simulink model "HybridEVModel"  (R2024b)
settings: Solver=ode45  StartTime=0.0  StopTime=421200  RelTol=1e-3
settings Model: Creator=zs  LastModifiedBy=zs
settings DataIOCC: SaveState=on

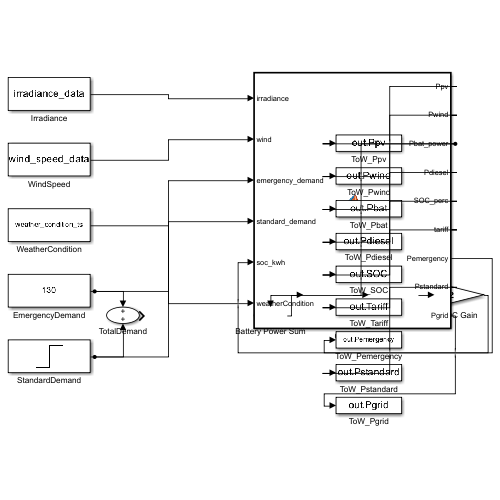
[thumbnail: Simulink's stored preview of the top-level diagram]
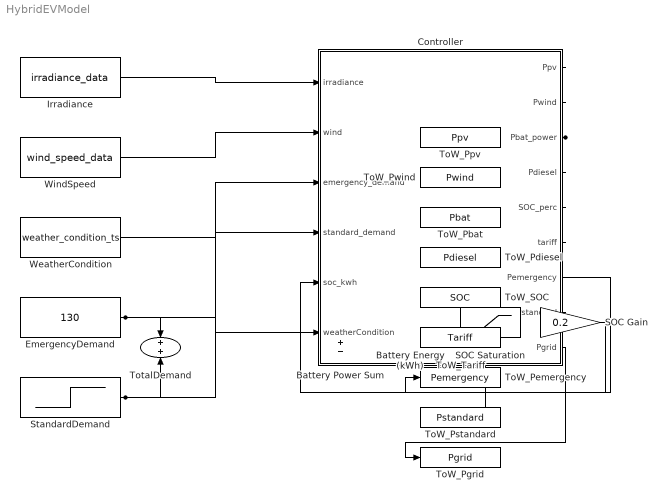
== system HybridEVModel ==
  Battery Energy (kWh) : Integrator  InitialCondition=250
  Battery Power Sum : Sum  Inputs=+-
  Controller : MATLAB Function  TreatAsAtomicUnit=on
  EmergencyDemand : Constant  Value=130
  Irradiance : FromWorkspace  VariableName=irradiance_data
  SOC Gain : Gain  Gain=0.2
  SOC Saturation : Saturate  UpperLimit=500  LowerLimit=0
  StandardDemand : Step  Time=28800  Before=1170  After=1170  SampleTime=0
  ToW_Pbat : ToWorkspace  VariableName=Pbat  SaveFormat=Timeseries  SampleTime=-1
  ToW_Pdiesel : ToWorkspace  VariableName=Pdiesel  SaveFormat=Timeseries  SampleTime=-1
  ToW_Pemergency : ToWorkspace  VariableName=Pemergency  SaveFormat=Timeseries  SampleTime=-1
  ToW_Pgrid : ToWorkspace  VariableName=Pgrid  SaveFormat=Timeseries  SampleTime=-1
  ToW_Ppv : ToWorkspace  VariableName=Ppv  SaveFormat=Timeseries  SampleTime=-1
  ToW_Pstandard : ToWorkspace  VariableName=Pstandard  SaveFormat=Timeseries  SampleTime=-1
  ToW_Pwind : ToWorkspace  VariableName=Pwind  SaveFormat=Timeseries  SampleTime=-1
  ToW_SOC : ToWorkspace  VariableName=SOC  SaveFormat=Timeseries  SampleTime=-1
  ToW_Tariff : ToWorkspace  VariableName=Tariff  SaveFormat=Timeseries  SampleTime=-1
  TotalDemand : Sum
  WeatherCondition : FromWorkspace  VariableName=weather_condition_ts
  WindSpeed : FromWorkspace  VariableName=wind_speed_data
  wires:
  Irradiance/1 -> Controller/1(irradiance)
  WindSpeed/1 -> Controller/2(wind)
  WeatherCondition/1 -> Controller/6(weatherCondition)
  EmergencyDemand/1 -> TotalDemand/1, Controller/3(emergency_demand)
  StandardDemand/1 -> TotalDemand/2, Controller/4(standard_demand)
  Controller/1(Ppv) -> ToW_Ppv/1
  Controller/2(Pwind) -> ToW_Pwind/1
  Controller/3(Pbat_power) -> ToW_Pbat/1, Battery Power Sum/1
  Controller/4(Pdiesel) -> ToW_Pdiesel/1
  Controller/5(SOC_perc) -> ToW_SOC/1
  Controller/6(tariff) -> ToW_Tariff/1
  Controller/7(Pemergency) -> ToW_Pemergency/1
  Controller/8(Pstandard) -> ToW_Pstandard/1
  Controller/9(Pgrid) -> ToW_Pgrid/1
  Battery Power Sum/1 -> Battery Energy (kWh)/1
  Battery Energy (kWh)/1 -> SOC Saturation/1
  SOC Saturation/1 -> SOC Gain/1
  SOC Gain/1 -> Controller/5(soc_kwh)

== matlab function HybridEVModel/Controller ==
  data: irradiance input; Ppv output; wind input; emergency_demand input; standard_demand input; soc_kwh input; weatherCondition input; Pwind output; Pbat_power output; Pdiesel output; SOC_perc output; tariff output; Pemergency output; Pstandard output; Pgrid output
function [Ppv, Pwind, Pbat_power, Pdiesel, SOC_perc, tariff, Pemergency, Pstandard, Pgrid] = fcn(irradiance, wind, emergency_demand, standard_demand, soc_kwh, weatherCondition)
Ppv = 0; Pwind = 0; Pbat_power = 0; Pdiesel = 0;
Pemergency = 0; Pstandard = 0; Pgrid = 0;
tariff = 0.30;
SOC_perc = 50;

panel_area = 300; solar_eff = 0.18;
rotor_diameter = 50; rho = 1.225; cp = 0.4;
rotor_area = pi * (rotor_diameter/2)^2;

if weatherCondition == 0
    solar_eff = solar_eff * 0.7;
    cp = cp * 0.8;
elseif weatherCondition == 2
    solar_eff = solar_eff * 1.2;
    cp = cp * 1.1;
end

Ppv = irradiance * panel_area * solar_eff / 1000;
Pwind = 0.5 * rho * rotor_area * (wind^3) * cp / 1000;
P_total = Ppv + Pwind;

battery_capacity = 500;
charge_eff = 0.95;
discharge_eff = 0.95;
diesel_min_soc = 0.2;

if P_total >= emergency_demand
    Pemergency = emergency_demand;
    excess = (P_total - emergency_demand) * charge_eff;
    soc_kwh = min(battery_capacity, soc_kwh + excess);
else
    Pemergency = P_total;
    remaining_emergency = emergency_demand - P_total;
    
    if soc_kwh >= remaining_emergency / discharge_eff
        Pemergency = Pemergency + remaining_emergency;
        soc_kwh = soc_kwh - (remaining_emergency / discharge_eff);
    else
        available_from_battery = soc_kwh * discharge_eff;
        Pemergency = Pemergency + available_from_battery;
        soc_kwh = 0;
        remaining_emergency = emergency_demand - Pemergency;
        
        if remaining_emergency > 0
            Pgrid = remaining_emergency;
            Pemergency = Pemergency + remaining_emergency;
        end
    end
end

remaining_gen = max(0, P_total - Pemergency);

if remaining_gen >= standard_demand
    Pstandard = standard_demand;
    excess = (remaining_gen - standard_demand) * charge_eff;
    soc_kwh = min(battery_capacity, soc_kwh + excess);
else
    Pstandard = remaining_gen;
    remaining_standard = standard_demand - remaining_gen;
    
    if soc_kwh >= remaining_standard / discharge_eff
        Pstandard = Pstandard + remaining_standard;
        soc_kwh = soc_kwh - (remaining_standard / discharge_eff);
    else
        available_from_battery = soc_kwh * discharge_eff;
        Pstandard = Pstandard + available_from_battery;
        soc_kwh = 0;
        remaining_standard = standard_demand - Pstandard;
        
        if weatherCondition == 0 && soc_kwh <= diesel_min_soc * battery_capacity
            Pdiesel = remaining_standard;
            Pstandard = Pstandard + remaining_standard;
        elseif remaining_standard > 0
            Pgrid = Pgrid + remaining_standard;
            Pstandard = Pstandard + remaining_standard;
        end
    end
end

Pbat_power = 0;

total_supplied = Pemergency + Pstandard;
if total_supplied > 0
    renewable_share = (min(P_total, total_supplied) / total_supplied) * 100;
else
    renewable_share = 0;
end

if renewable_share >= 75
    tariff = 0.15;
elseif renewable_share >= 50
    tariff = 0.225;
else
    tariff = 0.30;
end

SOC_perc = (soc_kwh / battery_capacity) * 100;
end
